simulink model "S2_surfs"  (R2025b)
settings: Solver=ode1be  StartTime=0.0  StopTime=0.5  RelTol=1e-3
values from neighbouring files (symbols this model uses):
  alpha1 = 0.5998    [S2_surf.m]
  alpha2 = 0.9989    [S2_surf.m]
  b11 = 0.9909    [S2_surf.m]
  b22 = 0.5998    [S2_surf.m]
  k1 = 15.0914    [S2_surf.m]
  k2 = 13.5948    [S2_surf.m]
undefined symbols (not defined in the file or in its folder): h, ks, magnitude, Mb
libraries: fod x12
settings Model: Creator=IT7  LastModifiedBy=Wassim DJ

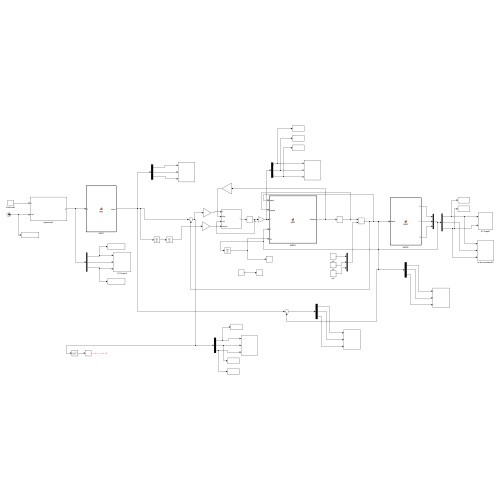
[thumbnail: Simulink's stored preview of the top-level diagram]
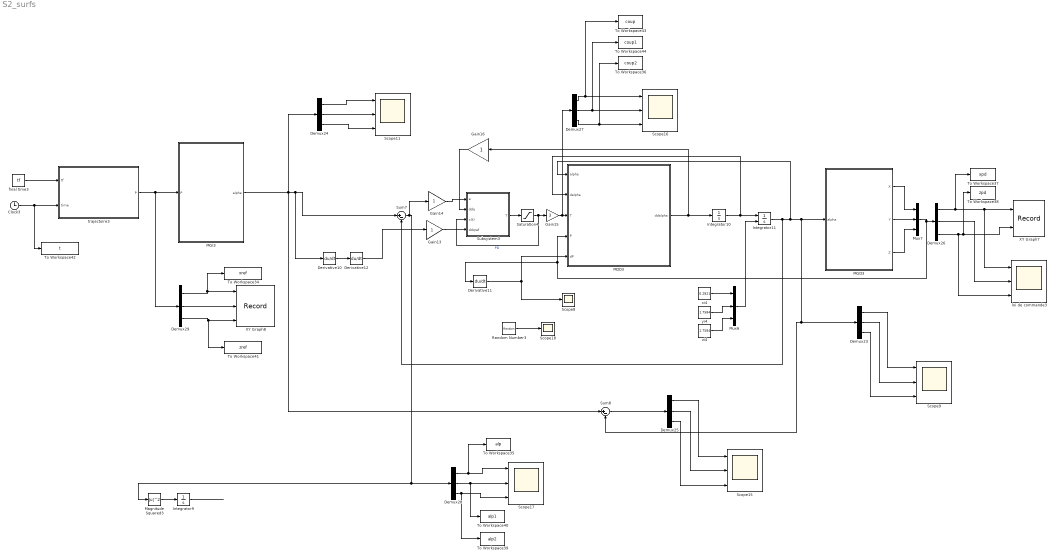
== system S2_surfs ==
  Clock3 : Clock
  Demux{23..29} (7 alike) : Demux  Outputs=3
  Derivative10 : Derivative
  Derivative11 : Derivative
  Derivative12 : Derivative
  Gain13 : Gain
  Gain14 : Gain
  Gain15 : Gain  Gain=3
  Gain16 : Gain
  Integrator10 : Integrator
  Integrator11 : Integrator  InitialConditionSource=external
  Integrator9 : Integrator
  MDD3 : MATLAB Function  TreatAsAtomicUnit=on
  MGD3 : MATLAB Function  TreatAsAtomicUnit=on
  MGI3 : MATLAB Function  TreatAsAtomicUnit=on
  Magnitude Squared3 : Math  Operator=magnitude^2
  Mux6 : Mux  Inputs=3
  Mux7 : Mux  Inputs=3
  Random Number3 : RandomNumber  Variance=0.001  Seed=4  SampleTime=0.001
  Saturation4 : Saturate  UpperLimit=15/12  LowerLimit=-15/12
  Scope{9,11,15..17} (5 alike) : Scope  NumInputPorts=3
      Scope11 settings: ActiveDisplayYMinimum=-0.0501  ActiveDisplayYMaximum=2.21858
      Scope15 settings: ActiveDisplayYMinimum=-0.0016  ActiveDisplayYMaximum=0.00114  DataLoggingVariableName=ScopeData2
      Scope16 settings: ActiveDisplayYMinimum=-18.75  ActiveDisplayYMaximum=18.75  DataLoggingVariableName=ScopeData3
      Scope17 settings: ActiveDisplayYMinimum=-0.00874  ActiveDisplayYMaximum=0.00356  DataLoggingVariableName=ScopeData4
      Scope9 settings: ActiveDisplayYMinimum=1.36342  ActiveDisplayYMaximum=5.69666  DataLoggingVariableName=ScopeData7
  Scope18 : Scope
      settings: ActiveDisplayYMinimum=-0.11225  ActiveDisplayYMaximum=0.1102  DataLoggingVariableName=ScopeData5
  Scope8 : Scope
      settings: ActiveDisplayYMinimum=-0.16191  ActiveDisplayYMaximum=10.52394  DataLoggingVariableName=ScopeData6
  Subsystem3 : Subsystem
  Sum7 : Sum  Inputs=|+-
  Sum8 : Sum  Inputs=|+-
  To Workspace34 : ToWorkspace  VariableName=xref  SampleTime=-1
      settings: Save2DSignal=2-D array (concatenate along first dimension)
  To Workspace35 : ToWorkspace  VariableName=alp  SampleTime=-1
      settings: Save2DSignal=2-D array (concatenate along first dimension)
  To Workspace36 : ToWorkspace  VariableName=coup2  SampleTime=-1
      settings: Save2DSignal=2-D array (concatenate along first dimension)
  To Workspace37 : ToWorkspace  VariableName=xpd  SampleTime=-1
      settings: Save2DSignal=2-D array (concatenate along first dimension)
  To Workspace38 : ToWorkspace  VariableName=zpd  SampleTime=-1
      settings: Save2DSignal=2-D array (concatenate along first dimension)
  To Workspace39 : ToWorkspace  VariableName=alp2  SampleTime=-1
      settings: Save2DSignal=2-D array (concatenate along first dimension)
  To Workspace40 : ToWorkspace  VariableName=alp1  SampleTime=-1
      settings: Save2DSignal=2-D array (concatenate along first dimension)
  To Workspace41 : ToWorkspace  VariableName=zref  SampleTime=-1
      settings: Save2DSignal=2-D array (concatenate along first dimension)
  To Workspace42 : ToWorkspace  VariableName=t  SampleTime=-1
      settings: Save2DSignal=2-D array (concatenate along first dimension)
  To Workspace43 : ToWorkspace  VariableName=coup  SampleTime=-1
      settings: Save2DSignal=2-D array (concatenate along first dimension)
  To Workspace44 : ToWorkspace  VariableName=coup1  SampleTime=-1
      settings: Save2DSignal=2-D array (concatenate along first dimension)
  XY Graph7 : Record  NumPorts=2.0  FileSettingsInternal="{\"entries\":[{\"content\":{\"excelSettings\":{\"content\":{},\"type\":\"Streamout.ExcelSettings\"},\"parquetSettings\":{\"content\":{},\"type\":\"Streamout.ParquetSettings\"}},\"type\":\"Streamout.FileSettingStorage\",\"uuid\":\"\"}],\"packageUris\":[\"http:\\/\\/schema.mathworks.com\\/mf0\\/streamout_blocks\\/R2020a\"],\"version\":\"1.0\"}"  FrameSettings=[0, 0]  Layout=[1 1]  SignalsInternal="{\"entries\":[{\"content\":{},\"type\":\"RecordBlkView.InputSignals\",\"uuid\":\"\"}],\"packageUris\":[\"http:\\/\\/schema.mathworks.com\\/mf0\\/streamout_blocks\\/R2020a\"],\"version\":\"1.0\"}"  VisualizationBindings="{\"xyplotplugin\":{\"info\":[{\"series\":[],\"subplotID\":1}]}}"  CompatibilityTag=XY  st=-1
  XY Graph8 : Record  NumPorts=3.0  FileSettingsInternal="{\"entries\":[{\"content\":{\"excelSettings\":{\"content\":{},\"type\":\"Streamout.ExcelSettings\"},\"parquetSettings\":{\"content\":{},\"type\":\"Streamout.ParquetSettings\"}},\"type\":\"Streamout.FileSettingStorage\",\"uuid\":\"\"}],\"packageUris\":[\"http:\\/\\/schema.mathworks.com\\/mf0\\/streamout_blocks\\/R2020a\"],\"version\":\"1.0\"}"  FrameSettings=[0, 0, 0]  Layout=[1 1]  SignalsInternal="{\"entries\":[{\"content\":{},\"type\":\"RecordBlkView.InputSignals\",\"uuid\":\"\"}],\"packageUris\":[\"http:\\/\\/schema.mathworks.com\\/mf0\\/streamout_blocks\\/R2020a\"],\"version\":\"1.0\"}"  VisualizationBindings="{\"xyplotplugin\":{\"info\":[{\"series\":[],\"subplotID\":1}]}}"  CompatibilityTag=XY  st=-1
  final time3 : Constant  Value=tf
  loi de commande3 : Scope  NumInputPorts=3
      settings: ActiveDisplayYMinimum=-0.50497  ActiveDisplayYMaximum=0.51496
  trajectoire3 : Subsystem
  xi4 : Constant  Value=0.2821
  yi4 : Constant  Value=1.7584
  zi4 : Constant  Value=1.7584
  wires:
  Integrator9/1 -> ?
  Demux26/3 -> loi de commande3/3, XY Graph7/2, To Workspace38/1
  Demux25/1 -> Scope15/1
  yi4/1 -> Mux6/2
  Mux6/1 -> Integrator11/2
  Demux28/3 -> To Workspace39/1, Scope17/3
  Demux24/2 -> Scope11/2
  MGI3/1(alpha) -> Derivative10/1, Sum7/1, Sum8/1, Demux24/1
  Demux25/2 -> Scope15/2
  Integrator11/1 -> Sum7/2, MDD3/1(alpha), MGD3/1(alpha), Demux23/1, Sum8/2
  Demux25/3 -> Scope15/3
  Gain13/1 -> Subsystem3/4(ddqref)
  Demux27/3 -> To Workspace36/1, Scope16/3
  Gain16/1 -> Subsystem3/2(ddq)
  MGD3/1(X) -> Mux7/1
  trajectoire3/1(P) -> Demux29/1, MGI3/1(P)
  MDD3/1(ddalpha) -> Gain16/1, Integrator10/1
  Demux23/3 -> Scope9/3
  zi4/1 -> Mux6/3
  Demux27/2 -> To Workspace44/1, Scope16/2
  MGD3/3(Z) -> Mux7/3
  Integrator10/1 -> MDD3/2(dalpha), Integrator11/1
  Demux23/2 -> Scope9/2
  Demux29/2 -> XY Graph8/2
  Sum7/1 -> Gain14/1, Magnitude Squared3/1, Demux28/1
  Demux23/1 -> Scope9/1
  Sum8/1 -> Demux25/1
  Mux7/1 -> MDD3/4(P), Derivative11/1, Demux26/1
  Gain15/1 -> Demux27/1, MDD3/3(T)
  Derivative10/1 -> Derivative12/1
  Demux24/1 -> Scope11/1
  MGD3/2(Y) -> Mux7/2
  Derivative11/1 -> MDD3/5(dP), Scope8/1
  xi4/1 -> Mux6/1
  Demux26/2 -> loi de commande3/2
  Demux27/1 -> To Workspace43/1, Scope16/1
  Clock3/1 -> To Workspace42/1, trajectoire3/2("time ")
  Demux28/1 -> To Workspace35/1, Scope17/1
  Random Number3/1 -> Scope18/1
  Demux29/1 -> To Workspace34/1, XY Graph8/1
  Demux24/3 -> Scope11/3
  Subsystem3/1(T) -> Saturation4/1
  Demux28/2 -> To Workspace40/1, Scope17/2
  final time3/1 -> trajectoire3/1(tf)
  Demux29/3 -> To Workspace41/1, XY Graph8/3
  Derivative12/1 -> Gain13/1
  Demux26/1 -> loi de commande3/1, XY Graph7/1, To Workspace37/1
  Magnitude Squared3/1 -> Integrator9/1
  Gain14/1 -> Subsystem3/1(e)
  Saturation4/1 -> Subsystem3/3(x(t)), Gain15/1  "PD"

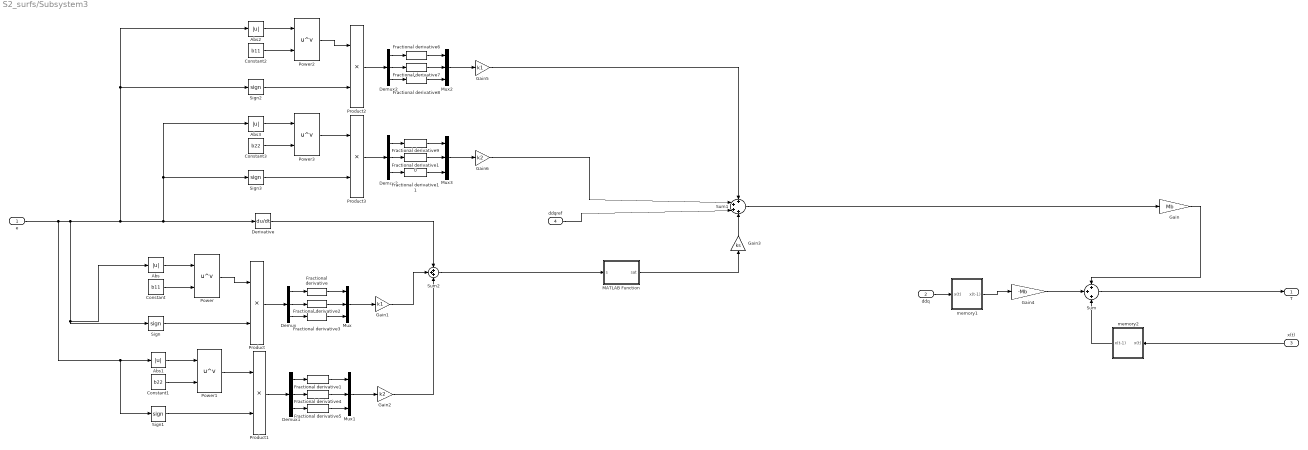
== system S2_surfs/Subsystem3 ==
  e : Inport
  ddq : Inport  Port=2
  x(t) : Inport  Port=3
  ddqref : Inport  Port=4
  Abs{,1..3} (4 alike) : Abs  SaturateOnIntegerOverflow=off
  Constant : Constant  Value=b11
  Constant1 : Constant  Value=b22
  Constant2 : Constant  Value=b11
  Constant3 : Constant  Value=b22
  Demux{,1..3} (4 alike) : Demux  Outputs=3
  Derivative : Derivative
  Fractional derivative : fod/Fractional derivative  gam=alpha1  ww=[0.001; 1000]  n=5  nFod=off
      settings: SourceProductName=FOMCON Toolbox
  Fractional derivative1 : fod/Fractional derivative  gam=alpha2 - 1  ww=[0.001; 1000]  n=5  nFod=off
      settings: SourceProductName=FOMCON Toolbox
  Fractional derivative10 : fod/Fractional derivative  gam=alpha2  ww=[0.001; 1000]  n=5  nFod=off
      settings: SourceProductName=FOMCON Toolbox
  Fractional derivative11 : fod/Fractional derivative  gam=alpha2  ww=[0.001; 1000]  n=5  nFod=off
      settings: SourceProductName=FOMCON Toolbox
  Fractional derivative2 : fod/Fractional derivative  gam=alpha1  ww=[0.001; 1000]  n=5  nFod=off
      settings: SourceProductName=FOMCON Toolbox
  Fractional derivative3 : fod/Fractional derivative  gam=alpha1  ww=[0.001; 1000]  n=5  nFod=off
      settings: SourceProductName=FOMCON Toolbox
  Fractional derivative4 : fod/Fractional derivative  gam=alpha2 - 1  ww=[0.001; 1000]  n=5  nFod=off
      settings: SourceProductName=FOMCON Toolbox
  Fractional derivative5 : fod/Fractional derivative  gam=alpha2 - 1  ww=[0.001; 1000]  n=5  nFod=off
      settings: SourceProductName=FOMCON Toolbox
  Fractional derivative6 : fod/Fractional derivative  gam=alpha1 + 1  ww=[0.001; 1000]  n=5  nFod=off
      settings: SourceProductName=FOMCON Toolbox
  Fractional derivative7 : fod/Fractional derivative  gam=alpha1 + 1  ww=[0.001; 1000]  n=5  nFod=off
      settings: SourceProductName=FOMCON Toolbox
  Fractional derivative8 : fod/Fractional derivative  gam=alpha1 + 1  ww=[0.001; 1000]  n=5  nFod=off
      settings: SourceProductName=FOMCON Toolbox
  Fractional derivative9 : fod/Fractional derivative  gam=alpha2  ww=[0.001; 1000]  n=5  nFod=off
      settings: SourceProductName=FOMCON Toolbox
  Gain : Gain  Gain=Mb
  Gain1 : Gain  Gain=k1
  Gain2 : Gain  Gain=k2
  Gain3 : Gain  Gain=ks
  Gain4 : Gain  Gain=-Mb
  Gain5 : Gain  Gain=k1
  Gain6 : Gain  Gain=k2
  MATLAB Function : MATLAB Function  TreatAsAtomicUnit=on
  Mux{,1..3} (4 alike) : Mux  Inputs=3
  Power{,1..3} (4 alike) : Math  Operator=pow
  Product{,1..3} (4 alike) : Product
  Sign{,1..3} (4 alike) : Signum
  Sum : Sum  Inputs=+++
  Sum1 : Sum  Inputs=++++
  Sum2 : Sum  Inputs=+++
  memory1 : Subsystem
  memory2 : Subsystem
  T : Outport  VectorParamsAs1DForOutWhenUnconnected=off
  wires:
  ddq/1 -> memory1/1(x(t))
  Sum1/1 -> Gain/1
  memory1/1(x(t-1)) -> Gain4/1
  Sum/1 -> T/1
  Gain/1 -> Sum/1
  Gain4/1 -> Sum/2
  memory2/1(x(t-1)) -> Sum/3
  x(t)/1 -> memory2/1(x(t))
  ddqref/1 -> Sum1/3
  Derivative/1 -> Sum2/1
  e/1 -> Sign1/1, Abs1/1, Derivative/1, Abs3/1, Sign3/1, Sign2/1, Abs2/1, Abs/1, Sign/1
  Abs/1 -> Power/1
  Constant/1 -> Power/2
  Sign/1 -> Product/2
  Power/1 -> Product/1
  Abs1/1 -> Power1/1
  Constant1/1 -> Power1/2
  Sign1/1 -> Product1/2
  Power1/1 -> Product1/1
  Gain1/1 -> Sum2/2
  Gain2/1 -> Sum2/3
  Product/1 -> Demux/1
  Demux/1 -> Fractional derivative/1
  Demux/2 -> Fractional derivative2/1
  Demux/3 -> Fractional derivative3/1
  Fractional derivative3/1 -> Mux/3
  Fractional derivative2/1 -> Mux/2
  Fractional derivative/1 -> Mux/1
  Mux/1 -> Gain1/1
  Mux1/1 -> Gain2/1
  Fractional derivative4/1 -> Mux1/2
  Fractional derivative1/1 -> Mux1/1
  Fractional derivative5/1 -> Mux1/3
  Demux1/2 -> Fractional derivative4/1
  Demux1/3 -> Fractional derivative5/1
  Demux1/1 -> Fractional derivative1/1
  Product1/1 -> Demux1/1
  Demux2/1 -> Fractional derivative6/1
  Demux2/3 -> Fractional derivative8/1
  Fractional derivative8/1 -> Mux2/3
  Mux2/1 -> Gain5/1
  Fractional derivative7/1 -> Mux2/2
  Fractional derivative6/1 -> Mux2/1
  Abs2/1 -> Power2/1
  Constant2/1 -> Power2/2
  Product2/1 -> Demux2/1
  Demux2/2 -> Fractional derivative7/1
  Sign2/1 -> Product2/2
  Power2/1 -> Product2/1
  Fractional derivative9/1 -> Mux3/1
  Demux3/3 -> Fractional derivative11/1
  Product3/1 -> Demux3/1
  Demux3/2 -> Fractional derivative10/1
  Constant3/1 -> Power3/2
  Sign3/1 -> Product3/2
  Demux3/1 -> Fractional derivative9/1
  Power3/1 -> Product3/1
  Fractional derivative10/1 -> Mux3/2
  Mux3/1 -> Gain6/1
  Abs3/1 -> Power3/1
  Fractional derivative11/1 -> Mux3/3
  Gain6/1 -> Sum1/2
  Gain5/1 -> Sum1/1
  Sum2/1 -> MATLAB Function/1(s)
  MATLAB Function/1(sat) -> Gain3/1
  Gain3/1 -> Sum1/4

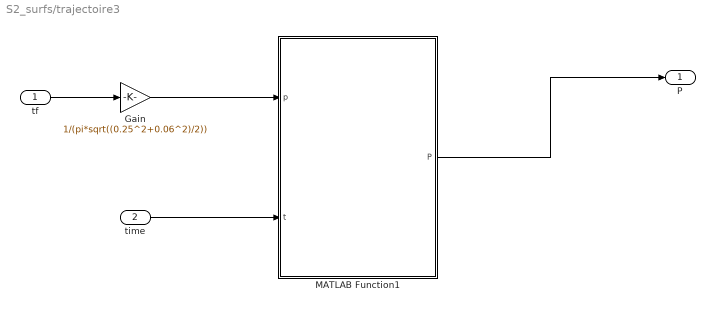
== system S2_surfs/trajectoire3 ==
  tf : Inport
  "time " : Inport  Port=2
  Gain : Gain  Gain=1/(pi*sqrt((0.25^2+0.06^2)/2))
  MATLAB Function1 : MATLAB Function  TreatAsAtomicUnit=on
  P : Outport  VectorParamsAs1DForOutWhenUnconnected=off
  wires:
  MATLAB Function1/1(P) -> P/1
  Gain/1 -> MATLAB Function1/1(p)
  "time "/1 -> MATLAB Function1/2(t)
  tf/1 -> Gain/1

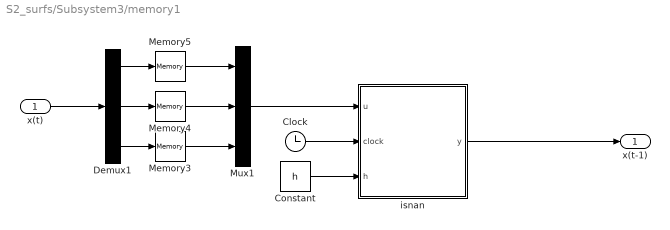
== system S2_surfs/Subsystem3/memory1 ==
  x(t) : Inport
  Clock : Clock
  Constant : Constant  Value=h
  Demux1 : Demux  Outputs=3
  Memory3 : Memory
  Memory4 : Memory
  Memory5 : Memory
  Mux1 : Mux  Inputs=3
  isnan : MATLAB Function  TreatAsAtomicUnit=on
  x(t-1) : Outport  VectorParamsAs1DForOutWhenUnconnected=off
  wires:
  x(t)/1 -> Demux1/1
  Demux1/1 -> Memory5/1
  Demux1/3 -> Memory3/1
  Demux1/2 -> Memory4/1
  Memory5/1 -> Mux1/1
  Memory4/1 -> Mux1/2
  Memory3/1 -> Mux1/3
  Mux1/1 -> isnan/1(u)
  isnan/1(y) -> x(t-1)/1
  Clock/1 -> isnan/2(clock)
  Constant/1 -> isnan/3(h)

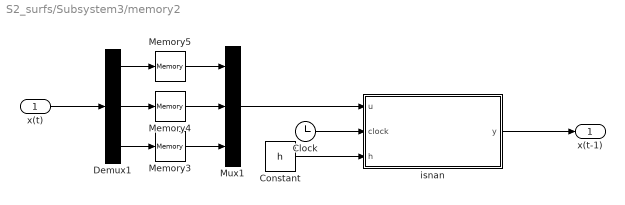
== system S2_surfs/Subsystem3/memory2 ==
  x(t) : Inport
  Clock : Clock
  Constant : Constant  Value=h
  Demux1 : Demux  Outputs=3
  Memory3 : Memory  InheritSampleTime=on
  Memory4 : Memory  InheritSampleTime=on
  Memory5 : Memory  InheritSampleTime=on
  Mux1 : Mux  Inputs=3
  isnan : MATLAB Function  TreatAsAtomicUnit=on
  x(t-1) : Outport  VectorParamsAs1DForOutWhenUnconnected=off
  wires:
  x(t)/1 -> Demux1/1
  Demux1/1 -> Memory5/1
  Demux1/3 -> Memory3/1
  Demux1/2 -> Memory4/1
  Memory5/1 -> Mux1/1
  Memory4/1 -> Mux1/2
  Memory3/1 -> Mux1/3
  Mux1/1 -> isnan/1(u)
  isnan/1(y) -> x(t-1)/1
  Clock/1 -> isnan/2(clock)
  Constant/1 -> isnan/3(h)

== matlab function S2_surfs/MDD3 ==
  data: alpha input; ddalpha output; dalpha input; T input; P input; dP input
function ddalpha  = MDD(alpha,dalpha,T,P,dP)
ddalpha = zeros(1,3);
phi = [0 2*pi/3 4*pi/3];
l1 = 0.205;
r = 0.15-0.024;
% these boudjedir table 2.1 page 30
mn = 0.042;
mfb = 0.028;
mb = 0.098;
mc = 0.015;
g = 9.81;
Im = 3.72e-5;
%mch=0.7;
% documentation 0
% rotation matrix
R1 = [cos(phi(1)) -sin(phi(1)) 0;sin(phi(1)) cos(phi(1)) 0;0 0 1];
R2 = [cos(phi(2)) -sin(phi(2)) 0;sin(phi(2)) cos(phi(2)) 0;0 0 1]; 
R3 = [cos(phi(3)) -sin(phi(3)) 0;sin(phi(3)) cos(phi(3)) 0;0 0 1]; 

% eq 4.4
s1 = [P(1);P(2);P(3)]-R1*([r;0;0]+[l1*cos(alpha(1));0;l1*sin(alpha(1))]);    
s2 = [P(1);P(2);P(3)]-R2*([r;0;0]+[l1*cos(alpha(2));0;l1*sin(alpha(2))]); 
s3 = [P(1);P(2);P(3)]-R3*([r;0;0]+[l1*cos(alpha(3));0;l1*sin(alpha(3))]); 

% eq 4.9
b1 = R1*[-l1*sin(alpha(1));0;l1*cos(alpha(1))];
b2 = R2*[-l1*sin(alpha(2));0;l1*cos(alpha(2))];
b3 = R3*[-l1*sin(alpha(3));0;l1*cos(alpha(3))];

% eq 4.8
ds1 = [dP(1);dP(2);dP(3)]-R1*[-l1*sin(alpha(1));0;l1*cos(alpha(1))]*dalpha(1);
ds2 = [dP(1);dP(2);dP(3)]-R2*[-l1*sin(alpha(2));0;l1*cos(alpha(2))]*dalpha(2);
ds3 = [dP(1);dP(2);dP(3)]-R3*[-l1*sin(alpha(3));0;l1*cos(alpha(3))]*dalpha(3);

db1 = R1*[-l1*cos(alpha(1));0;-l1*sin(alpha(1))]*dalpha(1);
db2 = R2*[-l1*cos(alpha(2));0;-l1*sin(alpha(2))]*dalpha(2);
db3 = R3*[-l1*cos(alpha(3));0;-l1*sin(alpha(3))]*dalpha(3);

% eq 4.13
J = inv([s1';s2';s3'])*[s1'*b1 0 0;0 s2'*b2 0;0 0 s3'*b3];

dJ = inv([s1';s2';s3'])*(-[ds1';ds2';ds3']*J+[ds1'*b1+s1'*db1 0 0;0 ds2'*b2+s2'*db2 0;0 0 ds3'*b3+s3'*db3]);
% these boudjedir
% equa 2.42
mnt = mn+mfb;  %+mch

% equa 2.49
Tgn = J'*mnt*[0 0 -g]';

% equa 2.44
mbr = mb+mc+2/3*mfb;

% equa 2.43
rgb = l1*(1/2*mb+mc+2/3*mfb)/mbr;

% equa 2.50
Tgb = rgb*mbr*g*[cos(alpha(1)) cos(alpha(2)) cos(alpha(3))]';

% equa 2.46
Ibc = l1^2*(mb/3+mc+2/3*mfb);
% equa 2.45
Ib = (Im*12^2+Ibc)*eye(3);

% equa 2.54
 ddalpha = (inv(Ib + mnt*J'*J)*(T - J'*mnt*dJ*dalpha' + Tgn + Tgb))';
if isnan(ddalpha)
    ddalpha = zeros(1,3);
end

== matlab function S2_surfs/MGD3 ==
  data: alpha input; X output; Y output; Z output
function [X,Y,Z]  = MGD(alpha)

phi = [0 2*pi/3 4*pi/3];
l1 = 0.205;
l2 = 0.380;
r = 0.15-0.024;

D = zeros(1,3);
E = zeros(1,3);
F = zeros(1,3);
G = zeros(1,3);

for i=1:3
   D(i)=-l2^2+l1^2+r^2+2*r*l1*cos(alpha(i));
   E(i)=2*(r+l1*cos(alpha(i)))*cos(phi(i));
   F(i)=2*(r+l1*cos(alpha(i)))*sin(phi(i));
   G(i)=-2*l1*sin(alpha(i))  ;
end
% H1 = -(E(3)-E(1))*(G(2)-G(1))+(G(3)-G(1))*(E(2)-E(1));
% H2 = -(F(3)-F(1))*(E(2)-E(1))+(E(3)-E(1))*(F(2)-F(1));
% H3 = -(D(3)-D(1))*(E(2)-E(1))+(E(3)-E(1))*(D(2)-D(1));
% H4 = (D(3)-D(1))*(F(2)-F(1))-(F(3)-F(1))*(D(1)-D(2));
% H5 = -(G(3)-G(1))*(F(2)-F(1))-(F(3)-F(1))*(G(1)-G(2));

H1 = E(1)*G(2)-E(1)*G(3)-E(2)*G(1)+E(2)*G(3)+E(3)*G(1)-E(3)*G(2);
H2 = E(1)*(-F(2)+F(3))+E(2)*(F(1)-F(3))+E(3)*(-F(1)+F(2));
H3 = E(1)*(-D(2)+D(3))+E(2)*(D(1)-D(3))+E(3)*(-D(1)+D(2));
H4 = F(1)*(D(2)-D(3))+F(2)*(-D(1)+D(3))+F(3)*(D(1)-D(2));
H5 = F(1)*(-G(2)+G(3))+F(2)*(G(1)-G(3))+F(3)*(-G(1)+G(2));

L = ((H5^2+H1^2)/(H2^2))+1;
M = 2*(H5*H4+H1*H3)/(H2^2)-(H5*E(1)+H1*F(1))/H2-G(1);
N = (H4^2+H3^2)/H2^2-(H4*E(1)+H3*F(1))/H2+D(1);
Z = min((-M+sqrt(abs(M^2-4*L*N)))/(2*L),(-M-sqrt(abs(M^2-4*L*N)))/(2*L));
X = Z*(H5/H2)+(H4/H2);
Y = Z*(H1/H2)+(H3/H2);

X = double(X);
Y = double(Y);
Z = double(Z);

== matlab function S2_surfs/MGI3 ==
  data: P input; alpha output
function alpha = MGI(P)
phi = [0 2*pi/3 4*pi/3];
l1 = 0.205;
l2 = 0.380;
r = 0.15-0.024;
X = P(1,1);
Y = P(1,2);
Z = P(1,3);

A = zeros(1,3);
B = 2*Z*l1;
C = zeros(1,3);

for i=1:3
A(i) = 2*r*l1-2*X*l1*cos(phi(i))-2*Y*l1*sin(phi(i));
C(i) = l2^2-l1^2-r^2-X^2-Y^2-Z^2+2*X*r*cos(phi(i))+2*Y*r*sin(phi(i));    
end

alpha = zeros(1,3);
for i=1:3
    alpha(i) =  2*atan( (2*B+sqrt(abs(4*B^2+4*(A(i)+C(i))*(A(i)-C(i)))))/(2*(A(i)+C(i))));
    alpha(i) = double(alpha(i));
end

== matlab function S2_surfs/Subsystem3/memory1/isnan ==
  data: u input; y output; clock input; h input
function y = fcn(u,clock,h)
y = zeros(length(u),1);
for i = 1:3
if isnan(u(i)) || clock/h < 3
    y(i) = 0; 
else 
   y(i) = u(i);
end
end

== matlab function S2_surfs/Subsystem3/memory2/isnan ==
  data: u input; y output; clock input; h input
function y = fcn(u,clock,h)
y = zeros(length(u),1);
for i = 1:3
if isnan(u(i)) || clock/h < 3
    y(i) = 0; 
else 
   y(i) = u(i);
end
end

== matlab function S2_surfs/trajectoire3/MATLAB Function1 ==
  data: P output; p input; t input
function P   = trajectoire(p,t)


A=0.25;
B=0.06;
D=pi*sqrt((A^2+B^2)/2);



Xdes=0.25-A*(1-cos(pi*(t)/(p*D)));
Ydes=0*t;
Zdes=-0.43+B*sin(pi*(t)/(p*D));

dXdes=-A*pi/(p*D)*(sin(pi*(t)/(p*D)));
dYdes=0*t;
dZdes=B*pi/(p*D)*cos(pi*(t)/(p*D));

ddXdes=A*pi/(p*D)*pi/(p*D)*cos(pi*(t)/(p*D));
ddYdes=0*t;
ddZdes=-B*pi/(p*D)*pi/(p*D)*sin(pi*(t)/(p*D));

% Xdes=-0.25+A*(1-cos(pi*t/(p*D)));
% Ydes=0*t;
% Zdes=-0.43+B*sin(pi*t/(p*D));

P = [Xdes,Ydes,Zdes];
%dP = [dXdes,dYdes,dZdes];
%ddP = [ddXdes,ddYdes,ddZdes];

end

== matlab function S2_surfs/Subsystem3/MATLAB Function ==
  data: s input; sat output
function sat = satuaration(s)
epsilon = 10;

if abs(s) < epsilon
    sat = s/epsilon;
else
    sat = sign(s);
end
